simulink model "Project_Mobius"  (R2023b)
settings: Solver=ode4  StartTime=0.0  StopTime=100  FixedStep=5e-3  RelTol=1e-3
values from neighbouring files (symbols this model uses):
  aileron_stuck = 0.1    [fault_insertion.m]
  aircraft_b = 2    [initial.m]
  aircraft_c = 0.275    [initial.m]
  aircraft_mass = 6.031    [initial.m]
  c1 = ((Iyy - Izz)*Izz - Ixz*Ixz)/sigma    (= -0.404494382022)    [initial.m]
  c2 = ((Ixx - Iyy + Izz)*Ixz)/sigma    (= 0)    [initial.m]
  c3 = Izz/sigma    (= 3.74531835206)    [initial.m]
  c4 = Ixz/sigma    (= 0)    [initial.m]
  c5 = (Izz - Ixx)/Iyy    (= 0.404494382022)    [initial.m]
  c6 = Ixz/Iyy    (= 0)    [initial.m]
  c7 = 1/Iyy    (= 3.74531835206)    [initial.m]
  c8 = (Ixx*(Ixx - Iyy) + Ixz*Ixz)/sigma    (= 0)    [initial.m]
  c9 = Ixx/sigma    (= 2.66666666667)    [initial.m]
  CD_fuselage = 0.027    [initial.m]
  CdDa = 0.092132    [initial.m]
  CdDe = 0.016043    [initial.m]
  CdDr = 0.0097403    [initial.m]
  CDmin = 0.06047    [initial.m]
  CL0 = 0.81857    [initial.m]
  CL_CDmin = 0.4806    [initial.m]
  CLa = 4.09127    [initial.m]
  CLa_dot = 0    [initial.m]
  Clb = -0.00161    [initial.m]
  ClDa = 0.286593    [initial.m]
  CLDa = -0.85291    [initial.m]
  CLDe = 0.50787    [initial.m]
  ClDr = 0.013407    [initial.m]
  Clp = -0.47584    [initial.m]
  CLq = 7.31097    [initial.m]
  Clr = 0.27153    [initial.m]
  Cm0 = 0.00763    [initial.m]
  Cma = -1.76966    [initial.m]
  CmDe = -1.83747    [initial.m]
  Cmq = -19.22663    [initial.m]
  Cnb = 0.0918    [initial.m]
  CnDa = 0.0049274    [initial.m]
  CnDr = -0.067036    [initial.m]
  Cnp = -0.13267    [initial.m]
  Cnr = -0.08829    [initial.m]
  CYb = -0.00157    [initial.m]
  CYDr = 0.128915    [initial.m]
  CYp = -0.00157    [initial.m]
  CYr = 0.18368    [initial.m]
  elevator_stuck = 0    [fault_insertion.m]
  fault_time_start = 1    [fault_insertion.m]
  flight_mode = 1    [initial.m]
  g = 9.8060    (= 9.806)    [initial.m]
  init_alpha = alpha_trim    (= 0)    [initial.m]
  init_h = 10    [initial.m]
  init_p = 0    [initial.m]
  init_phi = 0    [initial.m]
  init_psi = 0    [initial.m]
  init_q = 0    [initial.m]
  init_r = 0    [initial.m]
  init_theta = init_alpha    (= 0)    [initial.m]
  init_u = Vb(1)    [initial.m]
  init_v = Vb(2)    [initial.m]
  init_w = Vb(3)    [initial.m]
  init_x = 0    [initial.m]
  init_y = 0    [initial.m]
  K = 0.1328    [initial.m]
  Max_RPM = 10000    [initial.m]
  p_sensor_fault = 0    [fault_insertion.m]
  phi_sensor_fault = 0    [fault_insertion.m]
  PropDiameter = 0.3052    [initial.m]
  psi_sensor_fault = 0    [fault_insertion.m]
  q_sensor_fault = 0    [fault_insertion.m]
  r_sensor_fault = 0    [fault_insertion.m]
  rho = 1.2250    (= 1.225)    [initial.m]
  rotor1_direction = 1    [initial.m]
  rotor1_fail = 0    [fault_insertion.m]
  rotor2_direction = -1    [initial.m]
  rotor2_fail = 0    [fault_insertion.m]
  rotor3_direction = -1    [initial.m]
  rotor3_fail = 0    [fault_insertion.m]
  rotor4_direction = 1    [initial.m]
  rotor4_fail = 0    [fault_insertion.m]
  rotor_arm1 = [0.375,0.375,0]    [initial.m]
  rotor_arm2 = [0.375,-0.375,0]    [initial.m]
  rotor_arm3 = [-0.375,-0.375,0]    [initial.m]
  rotor_arm4 = [-0.375,0.375,0]    [initial.m]
  RPM1_init = rotor_n * 60    (= 5940)    [initial.m]
  RPM2_init = rotor_n * 60    (= 5940)    [initial.m]
  RPM3_init = 0    [initial.m]
  RPM4_init = 0    [initial.m]
  rudder_stuck = 0    [fault_insertion.m]
  theta_sensor_fault = 0    [fault_insertion.m]
  tilt1_fail = 0    [fault_insertion.m]
  tilt1_init = lambda    [initial.m]
  tilt2_fail = 0    [fault_insertion.m]
  tilt2_init = lambda    [initial.m]
  tilt3_init = 0    [initial.m]
  tilt4_init = 0    [initial.m]
  u_sensor_fault = 0    [fault_insertion.m]
  v_sensor_fault = 0    [fault_insertion.m]
  w_sensor_fault = 0    [fault_insertion.m]
undefined symbols (not defined in the file or in its folder): FixedWingMission, HoverMission
libraries: slpidlib x20, simulink_extras x12, simulink x7, aerolibasang x6, matrix_library x4, uavalgslib x4, sharedutil x1, sharedtransform x1
(part 1 of 4)
settings Model: Creator=admin  LastModifiedBy=admin

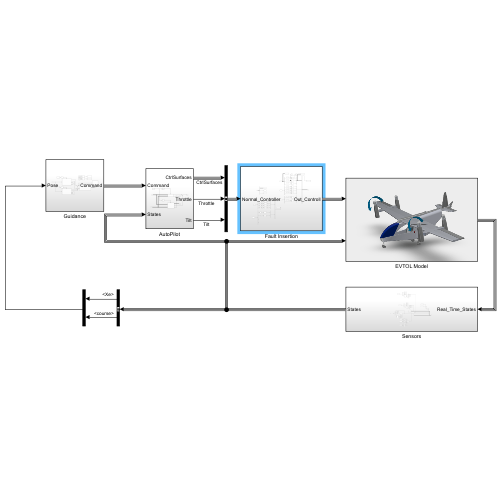
[thumbnail: Simulink's stored preview of the top-level diagram]
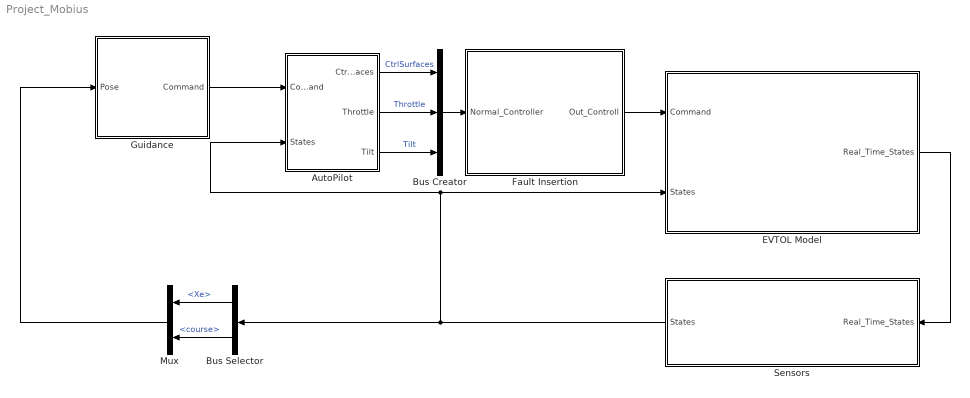
== system Project_Mobius ==
  AutoPilot : Subsystem
  Bus Creator : BusCreator  Inputs=3
  Bus Selector : BusSelector  OutputSignals=Xe,course
  EVTOL Model : Subsystem
      mask Display: image('EVTOL_Model.png');
  Fault Insertion : Subsystem
  Guidance : Subsystem
  Mux : Mux  Inputs=2
  Sensors : Subsystem
  wires:
  EVTOL Model/1(Real_Time_States) -> Sensors/1(Real_Time_States)
  Sensors/1(States) -> Bus Selector/1, AutoPilot/2(States), EVTOL Model/2(States)
  Bus Selector/1 -> Mux/1  "<Xe>"
  Bus Selector/2 -> Mux/2  "<course>"
  AutoPilot/1(CtrlSurfaces) -> Bus Creator/1  "CtrlSurfaces"
  AutoPilot/2(Throttle) -> Bus Creator/2  "Throttle"
  AutoPilot/3(Tilt) -> Bus Creator/3  "Tilt"
  Guidance/1(Command) -> AutoPilot/1(Command)
  Mux/1 -> Guidance/1(Pose)
  Bus Creator/1 -> Fault Insertion/1(Normal_Controller)
  Fault Insertion/1(Out_Controll) -> EVTOL Model/1(Command)

== system Project_Mobius/AutoPilot ==
  Command : Inport
  States : Inport  Port=2
  Compare To Constant : simulink/Logic and Bit Operations/Compare To Constant  relop===  const=0  OutDataTypeStr=boolean
  Compare To Constant1 : simulink/Logic and Bit Operations/Compare To Constant  relop===  const=1  OutDataTypeStr=boolean
  Constant : Constant  Value=flight_mode
  Fixed-Wing : Subsystem
  Multirotor : Subsystem
  Sum : Sum  Inputs=|++
  Sum1 : Sum  Inputs=|++
  CtrlSurfaces : Outport
  Throttle : Outport  Port=2
  Tilt : Outport  Port=3
  wires:
  Command/1 -> Fixed-Wing/1(Command), Multirotor/1(Command)
  States/1 -> Multirotor/2(States), Fixed-Wing/2(States)
  Constant/1 -> Compare To Constant1/1, Compare To Constant/1
  Compare To Constant/1 -> Multirotor/Enable
  Compare To Constant1/1 -> Fixed-Wing/Enable
  Fixed-Wing/1(CtrlSurfaces) -> CtrlSurfaces/1
  Sum/1 -> Throttle/1
  Multirotor/1(Throttle) -> Sum/1
  Fixed-Wing/3(Tilt) -> Sum1/2
  Multirotor/2(Tilt) -> Sum1/1
  Sum1/1 -> Tilt/1
  Fixed-Wing/2(Throttle) -> Sum/2

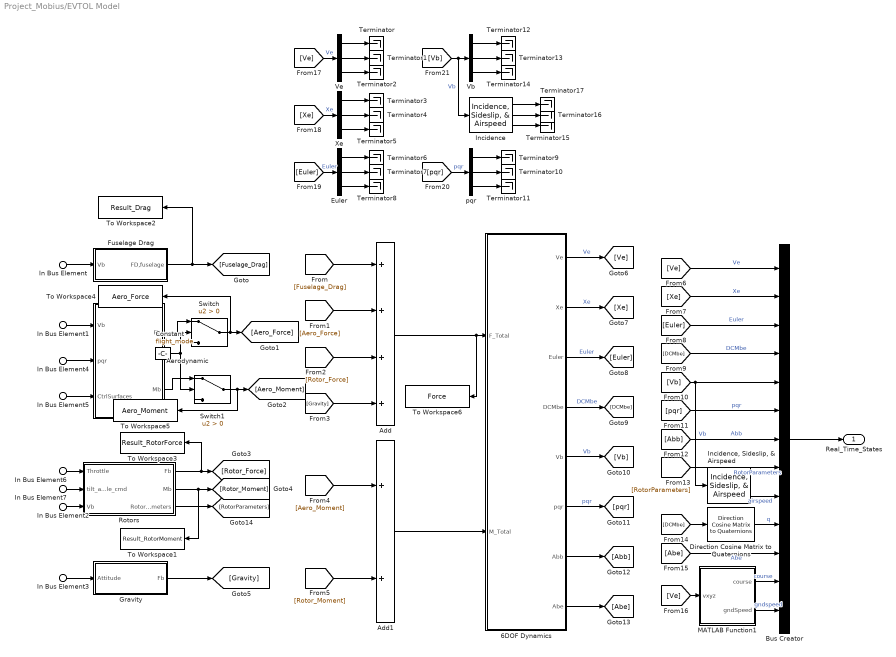
== system Project_Mobius/EVTOL Model ==
  In Bus Element5 : Inport  PortName=Command  Element=CtrlSurfaces
  In Bus Element6 : Inport  PortName=Command  Element=Throttle
  In Bus Element7 : Inport  PortName=Command  Element=Tilt
  In Bus Element : Inport  Port=2  PortName=States  Element=Vb
  In Bus Element1 : Inport  Port=2  PortName=States  Element=Vb
  In Bus Element2 : Inport  Port=2  PortName=States  Element=Vb
  In Bus Element3 : Inport  Port=2  PortName=States  Element=Euler
  In Bus Element4 : Inport  Port=2  PortName=States  Element=pqr
  6DOF Dynamics : Subsystem
  Add : Sum  Inputs=++++
  Add1 : Sum
  Aerodynamic : Subsystem
  Bus Creator : BusCreator  Inputs=13
  Constant : Constant  Value=flight_mode
  Direction Cosine Matrix to Quaternions : sharedtransform/Direction Cosine Matrix  to Quaternions  aMode=0  action=None  tolerance=eps(2)
      settings: LibrarySourceBlock=|
      | aerolibtransform2/Direction Cosine Matrix
      | to Quaternions
  Euler : Demux  Outputs=3
  Fuselage Drag : Subsystem
  Gravity : Subsystem
  Incidence : aerolibasang/Incidence, Sideslip, & Airspeed
  "Incidence, Sideslip, & Airspeed" : aerolibasang/Incidence, Sideslip, & Airspeed
  MATLAB Function1 : MATLAB Function  TreatAsAtomicUnit=on
  Rotors : Subsystem
  Switch : Switch  Criteria=u2 > Threshold  SaturateOnIntegerOverflow=off  InputSameDT=off
  Switch1 : Switch  Criteria=u2 > Threshold  SaturateOnIntegerOverflow=off  InputSameDT=off
  Terminator{,1..17} (18 alike) : Terminator
  To Workspace1 : ToWorkspace  VariableName=Result_RotorMoment  SampleTime=0.005
  To Workspace2 : ToWorkspace  VariableName=Result_Drag  SampleTime=0.005
  To Workspace3 : ToWorkspace  VariableName=Result_RotorForce  SampleTime=0.005
  To Workspace4 : ToWorkspace  VariableName=Aero_Force  SampleTime=0.005
  To Workspace5 : ToWorkspace  VariableName=Aero_Moment  SampleTime=0.005
  To Workspace6 : ToWorkspace  VariableName=Force  SampleTime=0.005
  Vb : Demux  Outputs=3
  Ve : Demux  Outputs=3
  Xe : Demux  Outputs=3
  pqr : Demux  Outputs=3
  Real_Time_States : Outport
  wires:
  [Rotor_Force] -> Add/3
  Fuselage Drag/1(FD,fuselage) -> To Workspace2/1, [Fuselage_Drag]
  [Rotor_Moment] -> Add1/2
  [Fuselage_Drag] -> Add/1
  Rotors/2(Mb) -> To Workspace1/1, [Rotor_Moment]
  [Aero_Moment] -> Add1/1
  [Aero_Force] -> Add/2
  [Gravity] -> Add/4
  Rotors/1(Fb) -> To Workspace3/1, [Rotor_Force]
  In Bus Element/1 -> Fuselage Drag/1(Vb)
  In Bus Element1/1 -> Aerodynamic/1(Vb)
  In Bus Element2/1 -> Rotors/3(Vb)
  In Bus Element3/1 -> Gravity/1(Attitude)
  In Bus Element4/1 -> Aerodynamic/2(pqr)
  Gravity/1(Fb) -> [Gravity]
  Bus Creator/1 -> Real_Time_States/1
  6DOF Dynamics/1(Ve) -> [Ve]  "Ve"
  6DOF Dynamics/2(Xe) -> [Xe]  "Xe"
  6DOF Dynamics/3(Euler) -> [Euler]  "Euler"
  6DOF Dynamics/4(DCMbe) -> [DCMbe]  "DCMbe"
  6DOF Dynamics/5(Vb) -> [Vb]  "Vb"
  6DOF Dynamics/6(pqr) -> [pqr]  "pqr"
  6DOF Dynamics/7(Abb) -> [Abb]
  6DOF Dynamics/8(Abe) -> [Abe]
  [Ve] -> Bus Creator/1  "Ve"
  [Xe] -> Bus Creator/2  "Xe"
  [Euler] -> Bus Creator/3  "Euler"
  [DCMbe] -> Bus Creator/4  "DCMbe"
  [Vb] -> Bus Creator/5, "Incidence, Sideslip, & Airspeed"/1  "Vb"
  [pqr] -> Bus Creator/6  "pqr"
  [Abb] -> Bus Creator/7  "Abb"
  [RotorParameters] -> Bus Creator/8  "RotorParameters"
  "Incidence, Sideslip, & Airspeed"/3 -> Bus Creator/9  "airspeed"
  Direction Cosine Matrix to Quaternions/1 -> Bus Creator/10  "q"
  [DCMbe] -> Direction Cosine Matrix to Quaternions/1
  [Abe] -> Bus Creator/11  "Abe"
  MATLAB Function1/1(course) -> Bus Creator/12  "course"
  MATLAB Function1/2(gndSpeed) -> Bus Creator/13  "gndspeed"
  [Ve] -> MATLAB Function1/1(vxyz)
  Rotors/3(RotorParameters) -> [RotorParameters]
  [Ve] -> Ve/1  "Ve"
  Ve/1 -> Terminator/1
  Ve/2 -> Terminator1/1
  Ve/3 -> Terminator2/1
  Xe/3 -> Terminator5/1
  Xe/1 -> Terminator3/1
  Xe/2 -> Terminator4/1
  [Xe] -> Xe/1  "Xe"
  [Euler] -> Euler/1  "Euler"
  Euler/1 -> Terminator6/1
  Euler/2 -> Terminator7/1
  Euler/3 -> Terminator8/1
  [pqr] -> pqr/1  "pqr"
  pqr/1 -> Terminator9/1
  pqr/2 -> Terminator10/1
  pqr/3 -> Terminator11/1
  Add1/1 -> 6DOF Dynamics/2(M_Total)
  Add/1 -> To Workspace6/1, 6DOF Dynamics/1(F_Total)
  Vb/1 -> Terminator12/1
  Vb/3 -> Terminator14/1
  [Vb] -> Incidence/1, Vb/1  "Vb"
  Vb/2 -> Terminator13/1
  Incidence/3 -> Terminator15/1
  Incidence/2 -> Terminator16/1
  Incidence/1 -> Terminator17/1
  In Bus Element5/1 -> Aerodynamic/3(CtrlSurfaces)
  In Bus Element6/1 -> Rotors/1(Throttle)
  In Bus Element7/1 -> Rotors/2(tilt_angle_cmd)
  Switch/1 -> To Workspace4/1, [Aero_Force]
  Aerodynamic/1(Fb) -> Switch/1
  Switch1/1 -> To Workspace5/1, [Aero_Moment]
  Constant/1 -> Switch1/2, Switch/2
  Aerodynamic/2(Mb) -> Switch1/1

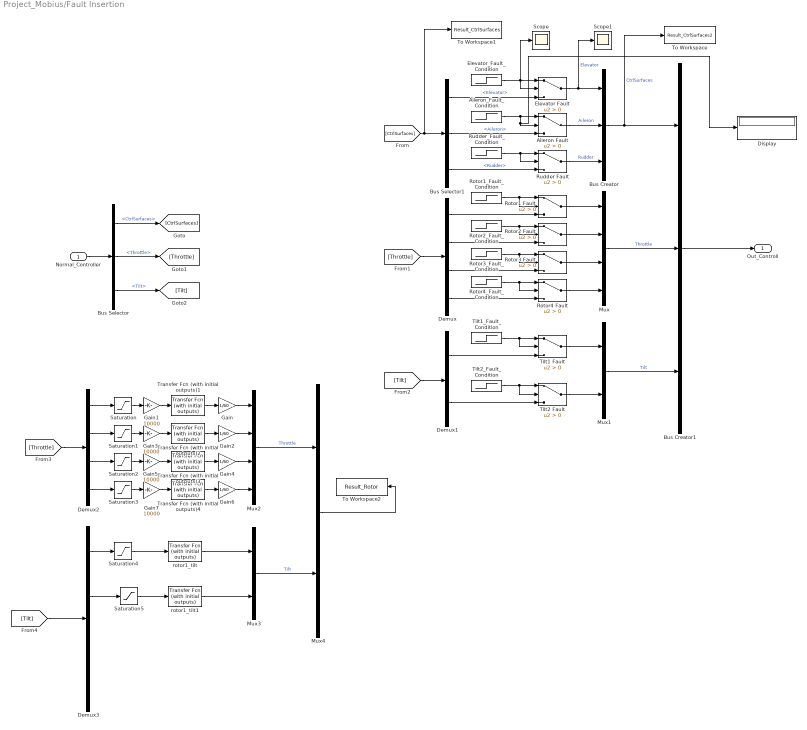
== system Project_Mobius/Fault Insertion ==
  Normal_Controller : Inport
  Aileron Fault : Switch  Criteria=u2 > Threshold  SaturateOnIntegerOverflow=off  InputSameDT=off
  Aileron_Fault_Condition : Step  Time=fault_time_start  After=aileron_stuck  SampleTime=0
  Bus Creator : BusCreator  Inputs=3
  Bus Creator1 : BusCreator  Inputs=3
  Bus Selector : BusSelector  OutputSignals=CtrlSurfaces,Throttle,Tilt
  Bus Selector1 : BusSelector  OutputSignals=Elevator,Aileron,Rudder
  Demux : Demux
  Demux1 : Demux  Outputs=2
  Demux2 : Demux
  Demux3 : Demux
  Display : Display
  Elevator Fault : Switch  Criteria=u2 > Threshold  SaturateOnIntegerOverflow=off  InputSameDT=off
  Elevator_Fault_Condition : Step  Time=fault_time_start  After=elevator_stuck  SampleTime=0
  Gain{,2,4,6} (4 alike) : Gain  Gain=1/60
  Gain{1,3,5,7} (4 alike) : Gain  Gain=10000
  Mux : Mux
  Mux1 : Mux  Inputs=2
  Mux2 : Mux
  Mux3 : Mux  Inputs=2
  Mux4 : Mux  Inputs=2
  Rotor1 Fault : Switch  Criteria=u2 > Threshold  SaturateOnIntegerOverflow=off  InputSameDT=off
  Rotor1_Fault_Condition : Step  Time=fault_time_start  After=rotor1_fail  SampleTime=0
  Rotor2 Fault : Switch  Criteria=u2 > Threshold  SaturateOnIntegerOverflow=off  InputSameDT=off
  Rotor2_Fault_Condition : Step  Time=fault_time_start  After=rotor2_fail  SampleTime=0
  Rotor3 Fault : Switch  Criteria=u2 > Threshold  SaturateOnIntegerOverflow=off  InputSameDT=off
  Rotor3_Fault_Condition : Step  Time=fault_time_start  After=rotor3_fail  SampleTime=0
  Rotor4 Fault : Switch  Criteria=u2 > Threshold  SaturateOnIntegerOverflow=off  InputSameDT=off
  Rotor4_Fault_Condition : Step  Time=fault_time_start  After=rotor4_fail  SampleTime=0
  Rudder Fault : Switch  Criteria=u2 > Threshold  SaturateOnIntegerOverflow=off  InputSameDT=off
  Rudder_Fault_Condition : Step  Time=fault_time_start  After=rudder_stuck  SampleTime=0
  Saturation{,1..3} (4 alike) : Saturate  UpperLimit=1  LowerLimit=0.1
  Saturation4 : Saturate  UpperLimit=90*pi/180  LowerLimit=-90*pi/180
  Saturation5 : Saturate  UpperLimit=90*pi/180  LowerLimit=-90*pi/180
  Scope : Scope
  Scope1 : Scope
  Tilt1 Fault : Switch  Criteria=u2 > Threshold  SaturateOnIntegerOverflow=off  InputSameDT=off
  Tilt1_Fault_Condition : Step  Time=fault_time_start  After=tilt1_fail  SampleTime=0
  Tilt2 Fault : Switch  Criteria=u2 > Threshold  SaturateOnIntegerOverflow=off  InputSameDT=off
  Tilt2_Fault_Condition : Step  Time=fault_time_start  After=tilt2_fail  SampleTime=0
  To Workspace : ToWorkspace  VariableName=Result_CtrlSurfaces2  SampleTime=-1
  To Workspace1 : ToWorkspace  VariableName=Result_CtrlSurfaces  SampleTime=-1
  To Workspace2 : ToWorkspace  VariableName=Result_Rotor  SampleTime=0.005
  Transfer Fcn (with initial outputs)1 : simulink_extras/Additional Linear/Transfer Fcn (with initial outputs)  N=[1]  D="[0.02  1]"  Y0=RPM1_init  U0=RPM1_init
  Transfer Fcn (with initial outputs)2 : simulink_extras/Additional Linear/Transfer Fcn (with initial outputs)  N=[1]  D="[0.02  1]"  Y0=RPM2_init  U0=RPM2_init
  Transfer Fcn (with initial outputs)3 : simulink_extras/Additional Linear/Transfer Fcn (with initial outputs)  N=[1]  D="[0.02  1]"  Y0=RPM3_init  U0=RPM3_init
  Transfer Fcn (with initial outputs)4 : simulink_extras/Additional Linear/Transfer Fcn (with initial outputs)  N=[1]  D="[0.02  1]"  Y0=RPM4_init  U0=RPM4_init
  rotor1_tilt : simulink_extras/Additional Linear/Transfer Fcn (with initial outputs)  N=[1]  D="[0.1  1]"  Y0=tilt1_init  U0=tilt1_init
  rotor1_tilt1 : simulink_extras/Additional Linear/Transfer Fcn (with initial outputs)  N=[1]  D="[0.1  1]"  Y0=tilt2_init  U0=tilt2_init
  Out_Controll : Outport
  wires:
  Normal_Controller/1 -> Bus Selector/1
  Bus Selector/1 -> [CtrlSurfaces]  "<CtrlSurfaces>"
  Bus Selector/2 -> [Throttle]  "<Throttle>"
  Bus Selector/3 -> [Tilt]  "<Tilt>"
  [CtrlSurfaces] -> To Workspace1/1, Bus Selector1/1
  Bus Selector1/1 -> Elevator Fault/3  "<Elevator>"
  Elevator_Fault_Condition/1 -> Scope/1, Elevator Fault/1, Elevator Fault/2
  Aileron_Fault_Condition/1 -> Aileron Fault/1, Display/1, Aileron Fault/2
  Bus Selector1/2 -> Aileron Fault/3  "<Aileron>"
  Bus Selector1/3 -> Rudder Fault/3  "<Rudder>"
  Rudder_Fault_Condition/1 -> Rudder Fault/1, Rudder Fault/2
  [Throttle] -> Demux/1
  Demux/1 -> Rotor1 Fault/3
  Rotor1_Fault_Condition/1 -> Rotor1 Fault/2, Rotor1 Fault/1
  Rotor2_Fault_Condition/1 -> Rotor2 Fault/2, Rotor2 Fault/1
  Demux/2 -> Rotor2 Fault/3
  Rotor3_Fault_Condition/1 -> Rotor3 Fault/2, Rotor3 Fault/1
  Demux/3 -> Rotor3 Fault/3
  Rotor4_Fault_Condition/1 -> Rotor4 Fault/2, Rotor4 Fault/1
  Demux/4 -> Rotor4 Fault/3
  [Tilt] -> Demux1/1
  Tilt1_Fault_Condition/1 -> Tilt1 Fault/2, Tilt1 Fault/1
  Demux1/1 -> Tilt1 Fault/3
  Tilt2_Fault_Condition/1 -> Tilt2 Fault/2, Tilt2 Fault/1
  Demux1/2 -> Tilt2 Fault/3
  Elevator Fault/1 -> Scope1/1, Bus Creator/1  "Elevator"
  Aileron Fault/1 -> Bus Creator/2  "Aileron"
  Rudder Fault/1 -> Bus Creator/3  "Rudder"
  Rotor1 Fault/1 -> Mux/1
  Rotor2 Fault/1 -> Mux/2
  Rotor3 Fault/1 -> Mux/3
  Rotor4 Fault/1 -> Mux/4
  Tilt1 Fault/1 -> Mux1/1
  Tilt2 Fault/1 -> Mux1/2
  Mux1/1 -> Bus Creator1/3  "Tilt"
  Mux/1 -> Bus Creator1/2  "Throttle"
  Bus Creator/1 -> To Workspace/1, Bus Creator1/1  "CtrlSurfaces"
  Bus Creator1/1 -> Out_Controll/1
  [Throttle] -> Demux2/1
  Demux2/1 -> Saturation/1
  Demux2/2 -> Saturation1/1
  Saturation1/1 -> Gain3/1
  Demux2/3 -> Saturation2/1
  Saturation2/1 -> Gain5/1
  Demux2/4 -> Saturation3/1
  Saturation3/1 -> Gain7/1
  [Tilt] -> Demux3/1
  Demux3/1 -> Saturation4/1
  Demux3/2 -> Saturation5/1
  Saturation4/1 -> rotor1_tilt/1
  Saturation5/1 -> rotor1_tilt1/1
  Mux3/1 -> Mux4/2  "Tilt"
  Mux4/1 -> To Workspace2/1
  Gain/1 -> Mux2/1
  Saturation/1 -> Gain1/1
  Gain1/1 -> Transfer Fcn (with initial outputs)1/1
  Transfer Fcn (with initial outputs)1/1 -> Gain/1
  Transfer Fcn (with initial outputs)2/1 -> Gain2/1
  Gain3/1 -> Transfer Fcn (with initial outputs)2/1
  Gain2/1 -> Mux2/2
  Transfer Fcn (with initial outputs)3/1 -> Gain4/1
  Gain5/1 -> Transfer Fcn (with initial outputs)3/1
  Gain4/1 -> Mux2/3
  Transfer Fcn (with initial outputs)4/1 -> Gain6/1
  Gain7/1 -> Transfer Fcn (with initial outputs)4/1
  Gain6/1 -> Mux2/4
  Mux2/1 -> Mux4/1  "Throttle"
  rotor1_tilt/1 -> Mux3/1
  rotor1_tilt1/1 -> Mux3/2

== system Project_Mobius/Guidance ==
  Pose : Inport
  Compare To Constant : simulink/Logic and Bit Operations/Compare To Constant  relop===  const=0  OutDataTypeStr=boolean
  Compare To Constant1 : simulink/Logic and Bit Operations/Compare To Constant  relop===  const=1  OutDataTypeStr=boolean
  Constant{,1..3} (4 alike) : Constant  Value=flight_mode
  Display : Display
  Fixed-Wing Mode : Subsystem
  Guidance Command : Subsystem
  MultiRotor Mode : Subsystem
  Sum : Sum  Inputs=|++
  Sum1 : Sum  Inputs=|++
  Switch : Switch  Criteria=u2 > Threshold  SaturateOnIntegerOverflow=off  InputSameDT=off
  Switch1 : Switch  Criteria=u2 > Threshold  SaturateOnIntegerOverflow=off  InputSameDT=off
  To Workspace : ToWorkspace  VariableName=mission_out  SampleTime=0.005
  To Workspace1 : ToWorkspace  VariableName=mission_done  SampleTime=0.005
  Command : Outport
  wires:
  Guidance Command/1(Command) -> Command/1
  Pose/1 -> MultiRotor Mode/1(Pose), Fixed-Wing Mode/1(Pose)
  Constant/1 -> Compare To Constant/1
  Compare To Constant/1 -> MultiRotor Mode/Enable
  Constant1/1 -> Compare To Constant1/1
  Compare To Constant1/1 -> Fixed-Wing Mode/Enable
  Sum/1 -> Display/1, Guidance Command/1(Desired Position)
  Sum1/1 -> Guidance Command/2(Desired_Course)
  Fixed-Wing Mode/1(Position_cmd) -> Sum/2
  MultiRotor Mode/1(Position_cmd) -> Sum/1
  MultiRotor Mode/2(Yaw_cmd) -> Sum1/1
  Fixed-Wing Mode/2(Yaw_cmd) -> Sum1/2
  Fixed-Wing Mode/3(Fix_mode) -> [Fix_mode]
  Fixed-Wing Mode/4(Fix_Mission_Done) -> [Fix_Mission_Done]
  MultiRotor Mode/3(Hover_mode) -> [Hover_mode]
  MultiRotor Mode/4(Hover_Mission_Done) -> [Hover_Mission_Done]
  Switch/1 -> To Workspace/1
  Switch1/1 -> To Workspace1/1
  Constant2/1 -> Switch/2
  Constant3/1 -> Switch1/2
  [Hover_mode] -> Switch/3
  [Fix_mode] -> Switch/1
  [Hover_Mission_Done] -> Switch1/3
  [Fix_Mission_Done] -> Switch1/1

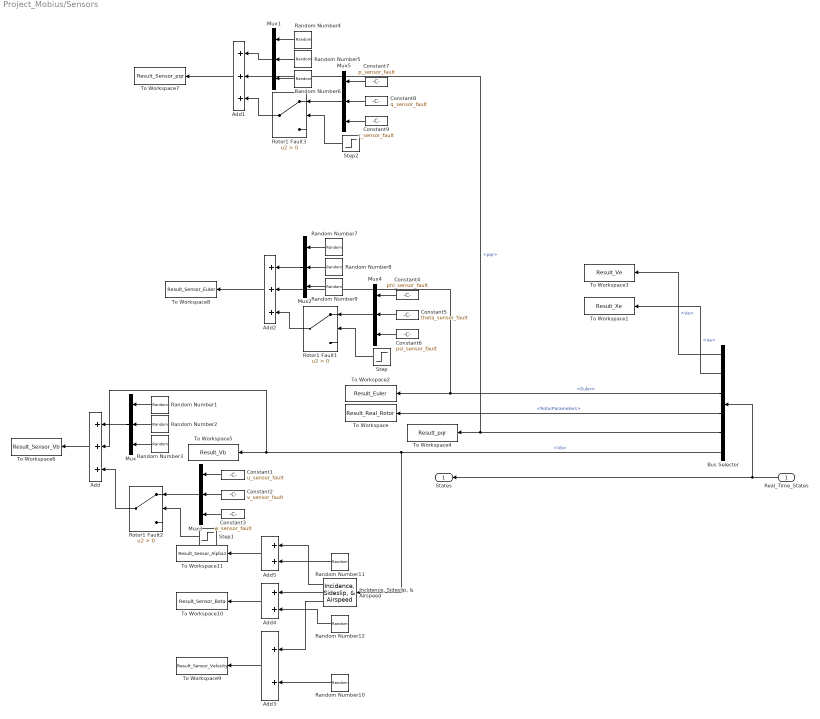
== system Project_Mobius/Sensors ==
  Real_Time_States : Inport
  Add : Sum  Inputs=+++
  Add1 : Sum  Inputs=+++
  Add2 : Sum  Inputs=+++
  Add3 : Sum
  Add4 : Sum
  Add5 : Sum
  Bus Selector : BusSelector  OutputSignals=Ve,Xe,Euler,RotorParameters,pqr,Vb
  Constant1 : Constant  Value=u_sensor_fault
  Constant2 : Constant  Value=v_sensor_fault
  Constant3 : Constant  Value=w_sensor_fault
  Constant4 : Constant  Value=phi_sensor_fault
  Constant5 : Constant  Value=theta_sensor_fault
  Constant6 : Constant  Value=psi_sensor_fault
  Constant7 : Constant  Value=p_sensor_fault  VectorParams1D=off
  Constant8 : Constant  Value=q_sensor_fault
  Constant9 : Constant  Value=r_sensor_fault
  "Incidence, Sideslip, & Airspeed" : aerolibasang/Incidence, Sideslip, & Airspeed
  Mux{,1..5} (6 alike) : Mux  Inputs=3
  Random Number{1..3,10} (4 alike) : RandomNumber  Variance=9e-4  SampleTime=5e-3
  Random Number11 : RandomNumber  Variance=9e-6  SampleTime=5e-3
  Random Number12 : RandomNumber  Variance=9e-6  SampleTime=5e-3
  Random Number4 : RandomNumber  Variance=(0.01)*(0.01)  SampleTime=5e-3
  Random Number5 : RandomNumber  Variance=(0.01)*(0.01)  SampleTime=5e-3
  Random Number6 : RandomNumber  Variance=(0.01)*(0.01)  SampleTime=5e-3
  Random Number7 : RandomNumber  Variance=(0.07*pi/180/3)^2  SampleTime=5e-3
  Random Number8 : RandomNumber  Variance=(0.07*pi/180/3)^2  SampleTime=5e-3
  Random Number9 : RandomNumber  Variance=(0.07*pi/180/3)^2  SampleTime=5e-3
  Rotor1 Fault1 : Switch  Criteria=u2 > Threshold  SaturateOnIntegerOverflow=off  InputSameDT=off
  Rotor1 Fault2 : Switch  Criteria=u2 > Threshold  SaturateOnIntegerOverflow=off  InputSameDT=off
  Rotor1 Fault3 : Switch  Criteria=u2 > Threshold  SaturateOnIntegerOverflow=off  InputSameDT=off
  Step : Step  Time=fault_time_start  SampleTime=0
  Step1 : Step  Time=fault_time_start  SampleTime=0
  Step2 : Step  Time=fault_time_start  SampleTime=0
  To Workspace : ToWorkspace  VariableName=Result_Real_Rotor  SampleTime=0.005
  To Workspace1 : ToWorkspace  VariableName=Result_Xe  SampleTime=0.005
  To Workspace10 : ToWorkspace  VariableName=Result_Sensor_Beta  SampleTime=0.005
  To Workspace11 : ToWorkspace  VariableName=Result_Sensor_Alpha1  SampleTime=0.005
  To Workspace2 : ToWorkspace  VariableName=Result_Euler  SampleTime=0.005
  To Workspace3 : ToWorkspace  VariableName=Result_Ve  SampleTime=0.005
  To Workspace4 : ToWorkspace  VariableName=Result_pqr  SampleTime=0.005
  To Workspace5 : ToWorkspace  VariableName=Result_Vb  SampleTime=0.005
  To Workspace6 : ToWorkspace  VariableName=Result_Sensor_Vb  SampleTime=0.005
  To Workspace7 : ToWorkspace  VariableName=Result_Sensor_pqr  SampleTime=0.005
  To Workspace8 : ToWorkspace  VariableName=Result_Sensor_Euler  SampleTime=0.005
  To Workspace9 : ToWorkspace  VariableName=Result_Sensor_Velocity  SampleTime=0.005
  States : Outport
  wires:
  Real_Time_States/1 -> Bus Selector/1, States/1
  Bus Selector/1 -> To Workspace3/1  "<Ve>"
  Bus Selector/2 -> To Workspace1/1  "<Xe>"
  Bus Selector/4 -> To Workspace/1  "<RotorParameters>"
  Bus Selector/6 -> "Incidence, Sideslip, & Airspeed"/1, Add/2, To Workspace5/1  "<Vb>"
  Random Number1/1 -> Mux/1
  Random Number2/1 -> Mux/2
  Random Number3/1 -> Mux/3
  Mux/1 -> Add/1
  Add/1 -> To Workspace6/1
  Random Number5/1 -> Mux1/2
  Bus Selector/5 -> To Workspace4/1, Add1/2  "<pqr>"
  Random Number6/1 -> Mux1/3
  Random Number4/1 -> Mux1/1
  Add1/1 -> To Workspace7/1
  Mux1/1 -> Add1/1
  Add2/1 -> To Workspace8/1
  Random Number7/1 -> Mux2/1
  Random Number8/1 -> Mux2/2
  Bus Selector/3 -> Add2/2, To Workspace2/1  "<Euler>"
  Mux2/1 -> Add2/1
  Random Number9/1 -> Mux2/3
  Constant4/1 -> Mux4/1
  Constant5/1 -> Mux4/2
  Constant6/1 -> Mux4/3
  Mux4/1 -> Rotor1 Fault1/1
  Rotor1 Fault1/1 -> Add2/3
  Step/1 -> Rotor1 Fault1/2
  Step1/1 -> Rotor1 Fault2/2
  Constant1/1 -> Mux3/1
  Constant2/1 -> Mux3/2
  Constant3/1 -> Mux3/3
  Mux3/1 -> Rotor1 Fault2/1
  Rotor1 Fault2/1 -> Add/3
  Mux5/1 -> Rotor1 Fault3/1
  Rotor1 Fault3/1 -> Add1/3
  Constant8/1 -> Mux5/2
  Constant9/1 -> Mux5/3
  Step2/1 -> Rotor1 Fault3/2
  Constant7/1 -> Mux5/1
  "Incidence, Sideslip, & Airspeed"/3 -> Add3/1
  Random Number10/1 -> Add3/2
  Add3/1 -> To Workspace9/1
  "Incidence, Sideslip, & Airspeed"/2 -> Add4/1
  Add4/1 -> To Workspace10/1
  "Incidence, Sideslip, & Airspeed"/1 -> Add5/1
  Add5/1 -> To Workspace11/1
  Random Number11/1 -> Add5/2
  Random Number12/1 -> Add4/2

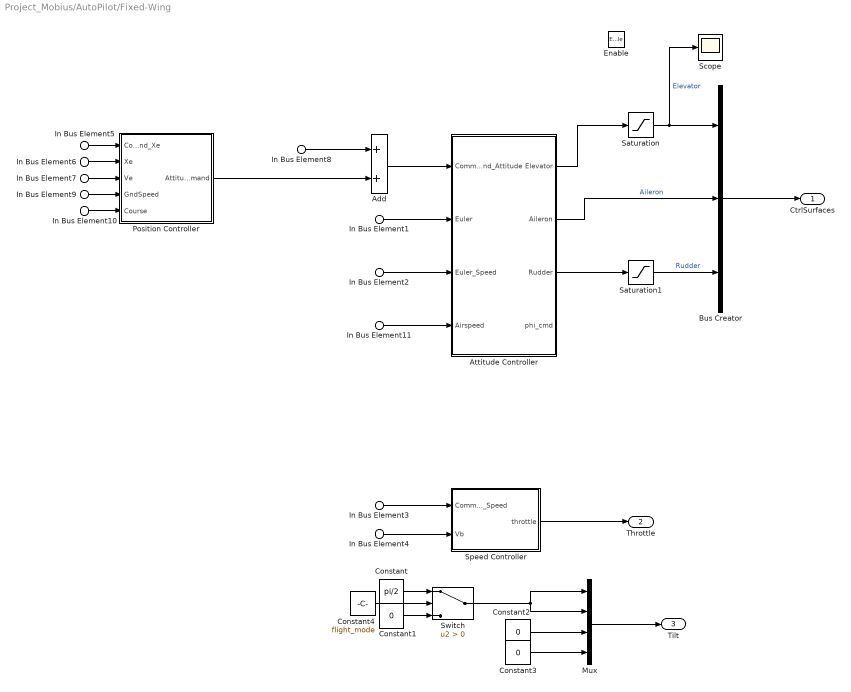
== system Project_Mobius/AutoPilot/Fixed-Wing ==
  In Bus Element3 : Inport  PortName=Command  Element=Speed
  In Bus Element5 : Inport  PortName=Command  Element=Xe
  In Bus Element8 : Inport  PortName=Command  Element=Attitude
  In Bus Element1 : Inport  Port=2  PortName=States  Element=Euler
  In Bus Element2 : Inport  Port=2  PortName=States  Element=pqr
  In Bus Element4 : Inport  Port=2  PortName=States  Element=Vb
  In Bus Element6 : Inport  Port=2  PortName=States  Element=Xe
  In Bus Element7 : Inport  Port=2  PortName=States  Element=Ve
  In Bus Element9 : Inport  Port=2  PortName=States  Element=gndspeed
  In Bus Element10 : Inport  Port=2  PortName=States  Element=course
  In Bus Element11 : Inport  Port=2  PortName=States  Element=airspeed
  Enable : EnablePort
  Add : Sum
  Attitude Controller : Subsystem
  Bus Creator : BusCreator  Inputs=3
  Constant : Constant  Value=pi/2
  Constant1 : Constant  Value=0
  Constant2 : Constant  Value=0
  Constant3 : Constant  Value=0
  Constant4 : Constant  Value=flight_mode
  Mux : Mux
  Position Controller : Subsystem
  Saturation : Saturate  UpperLimit=20*pi/180  LowerLimit=-20*pi/180
  Saturation1 : Saturate  UpperLimit=30*pi/180  LowerLimit=-30*pi/180
  Scope : Scope
  Speed Controller : Subsystem
  Switch : Switch  Criteria=u2 > Threshold  SaturateOnIntegerOverflow=off  InputSameDT=off
  CtrlSurfaces : Outport
  Throttle : Outport  Port=2
  Tilt : Outport  Port=3
  wires:
  In Bus Element1/1 -> Attitude Controller/2(Euler)
  In Bus Element2/1 -> Attitude Controller/3(Euler_Speed)
  Attitude Controller/1(Elevator) -> Saturation/1
  Attitude Controller/2(Aileron) -> Bus Creator/2  "Aileron"
  Attitude Controller/3(Rudder) -> Saturation1/1
  Bus Creator/1 -> CtrlSurfaces/1
  In Bus Element3/1 -> Speed Controller/1(Command_Speed)
  In Bus Element4/1 -> Speed Controller/2(Vb)
  In Bus Element5/1 -> Position Controller/1(Command_Xe)
  In Bus Element6/1 -> Position Controller/2(Xe)
  In Bus Element7/1 -> Position Controller/3(Ve)
  Position Controller/1(Attitude_command) -> Add/2
  Add/1 -> Attitude Controller/1(Command_Attitude)
  In Bus Element8/1 -> Add/1
  Saturation/1 -> Scope/1, Bus Creator/1  "Elevator"
  In Bus Element9/1 -> Position Controller/4(GndSpeed)
  In Bus Element10/1 -> Position Controller/5(Course)
  Saturation1/1 -> Bus Creator/3  "Rudder"
  In Bus Element11/1 -> Attitude Controller/4(Airspeed)
  Constant2/1 -> Mux/3
  Constant3/1 -> Mux/4
  Mux/1 -> Tilt/1
  Constant4/1 -> Switch/2
  Constant/1 -> Switch/1
  Constant1/1 -> Switch/3
  Switch/1 -> Mux/1, Mux/2
  Speed Controller/1(throttle) -> Throttle/1
